simulink model "template_KR3_PreRTHS"  (Simulink 7.9)
settings: Solver=FixedStepDiscrete  StartTime=0.0  StopTime=RunningTime  FixedStep=sample  RelTol=1e-3
undefined symbols (not defined in the file): ElementsStruct, Integrator, NumFreeDOF, RigidLinkMasterMatrix, RigidLinkNo, RigidLinkNodeID, RigidLinkSlaveMatrix, sample, SampleRate, Structure
libraries: HybridFEMLibrary x1
(part 2 of 2)

== matlab function EffForcePrevStep/MATLAB Function ==
  data: MassMatrixHat2 input double; Acceleration input double; DampingMatrixFree input double; Velocity input double; Alphaf input double; RestoringForce input double; EffForcePrevStep output double; EQScaleFactor input double; PEFF input double
function EffForcePrevStep   = fcn(MassMatrixHat2,...
                                Acceleration,...
                                DampingMatrixFree,...
                                Velocity,...
                                Alphaf,...
                                RestoringForce,...                                
                                EQScaleFactor,...
                                PEFF)

EffForcePrevStep = MassMatrixHat2 * Acceleration + ...
                DampingMatrixFree * Velocity + Alphaf * ...
                (RestoringForce - EQScaleFactor * PEFF);
